simulink model "DSB_TC_Receiver_Part_3_2"  (R2022a)
settings: Solver=FixedStepDiscrete  StartTime=0.0  StopTime=inf  RelTol=1e-3
PreLoadFcn:
  | addpath('matlab/DSB_TC');
libraries: matrix_library x2, dspsnks4 x1, dspvision x1, dspsigops x1
settings Model: Creator=vovan  LastModifiedBy=vovan

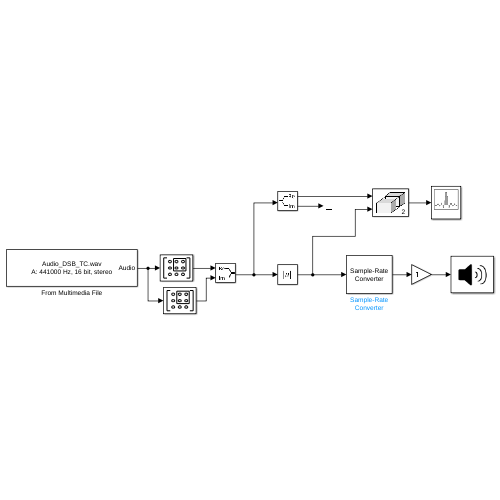
[thumbnail: Simulink's stored preview of the top-level diagram]
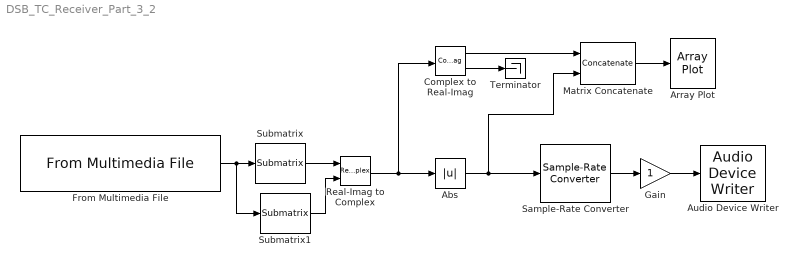
== system DSB_TC_Receiver_Part_3_2 ==
  Abs : Abs  SaturateOnIntegerOverflow=off
  Array Plot : ArrayPlot  WindowPosition=[560.000000,290.000000,800.000000,500.000000,]  Visible=on  ScopeFrameLocation=window  PlotType=Line  AxesScaling=Manual  YLimits=[-1,1]  ShowLegend=on
  Audio Device Writer : dspsnks4/Audio Device Writer  Driver=ALSA  Device=Default  InheritSampleRate=on  SampleRate=44100  BitDepth=16-bit integer  BufferSize=4096  NumBuffers=10  DefaultOutputChannelMapping=on  OutputChannelMapping=1:2  OutputNumUnderrunSamples=off  DriverIdx=8  DeviceWarnFlag=''
  Complex to Real-Imag : ComplexToRealImag
  From Multimedia File : dspvision/From Multimedia File  inputFilename=wav/Audio_DSB_TC.wav  readRange=[1 Inf]  loop=on  numPlays=inf  outputStreams=Audio only  videoDataType=single  audioDataType=double  inheritSampleTime=on  userDefinedSampleTime=1/30  noAudioOutput=off  isIntensityVideo=off  fourcc=RGB  colorVideoFormat=Separate color signals  outputEOF=off  dataOrg=Column-major  audioFrameSize=10000  computeAudioFrameSize=off  outSamplingMode=Sample based
  Gain : Gain
  Matrix Concatenate : Concatenate  Mode=Multidimensional array  ConcatenateDimension=2
  Real-Imag to Complex : RealImagToComplex
  Sample-Rate Converter : dspsigops/Sample-Rate Converter  InputSampleRate=441000  OutputSampleRate=44100  OutputRateTolerance=0  Bandwidth=40e3  StopbandAttenuation=80  SimulateUsing=Code generation
      settings: SourceProductBaseCode=DS
  Submatrix : matrix_library/Submatrix  RowSpan=All rows  RowStartMode=First  RowStartIndex=1  RowEndMode=Last  RowEndIndex=1  ColSpan=Range of columns  ColStartMode=First  ColStartIndex=1  ColEndMode=Index  ColEndIndex=1
      settings: SourceProductBaseCode=SL
  Submatrix1 : matrix_library/Submatrix  RowSpan=All rows  RowStartMode=First  RowStartIndex=1  RowEndMode=Last  RowEndIndex=1  ColSpan=Range of columns  ColStartMode=Last  ColStartIndex=1  ColEndMode=Index  ColEndIndex=1
      settings: SourceProductBaseCode=SL
  Terminator : Terminator
  wires:
  From Multimedia File/1 -> Submatrix1/1, Submatrix/1
  Submatrix/1 -> Real-Imag to Complex/1
  Submatrix1/1 -> Real-Imag to Complex/2
  Sample-Rate Converter/1 -> Gain/1
  Abs/1 -> Sample-Rate Converter/1, Matrix Concatenate/2
  Gain/1 -> Audio Device Writer/1
  Matrix Concatenate/1 -> Array Plot/1
  Real-Imag to Complex/1 -> Complex to Real-Imag/1, Abs/1
  Complex to Real-Imag/2 -> Terminator/1
  Complex to Real-Imag/1 -> Matrix Concatenate/1
